simulink model "model_fitting"  (R2019a)
settings: Solver=ode2  StartTime=0.0  StopTime=200  FixedStep=0.1  RelTol=1e-3
settings Model: Creator=HP  LastModifiedBy=swastik
settings DataIOCC: ReturnWorkspaceOutputs=off
settings DebuggingCC: ArithmeticOperatorsInVariantConditions=warning

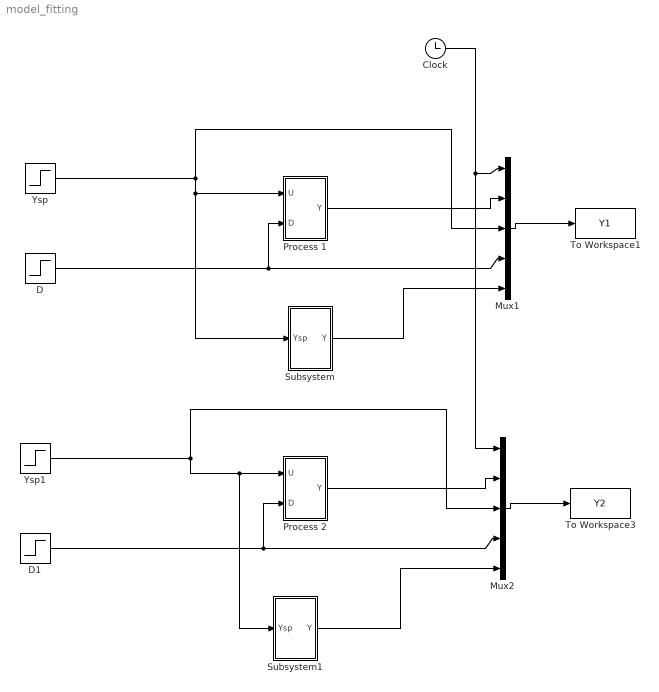
== system model_fitting ==
  Clock : Clock
  D : Step  Time=0  After=0  SampleTime=0
  D1 : Step  Time=0  After=0  SampleTime=0
  Mux1 : Mux  Inputs=5
  Mux2 : Mux  Inputs=5
  Process 1 : Subsystem
  Process 2 : Subsystem
  Subsystem : Subsystem  mask{Km=1.9991, Tm=16.6899, D=23.3484}
      mask prompts: Km "Gain"; Tm "lag"; D "dead time"
  Subsystem1 : Subsystem  mask{K=0.9992, T1=11.25, T2=11.25, T3=15.25, D=16}
      mask prompts: K "Gain1"; T1 "lag1"; T2 "lag2"; T3 "lead"; D "dead time"
  To Workspace1 : ToWorkspace  VariableName=Y1  SampleTime=-1
  To Workspace3 : ToWorkspace  VariableName=Y2  SampleTime=-1
  Ysp : Step  Time=0  SampleTime=0
  Ysp1 : Step  Time=0  SampleTime=0
  wires:
  Mux1/1 -> To Workspace1/1
  Clock/1 -> Mux1/1, Mux2/1
  Ysp/1 -> Subsystem/1(Ysp), Process 1/1(U), Mux1/3
  Process 1/1(Y) -> Mux1/2
  D/1 -> Mux1/4, Process 1/2(D)
  Mux2/1 -> To Workspace3/1
  Ysp1/1 -> Process 2/1(U), Subsystem1/1(Ysp), Mux2/3
  Process 2/1(Y) -> Mux2/2
  D1/1 -> Process 2/2(D), Mux2/4
  Subsystem/1(Y) -> Mux1/5
  Subsystem1/1(Y) -> Mux2/5

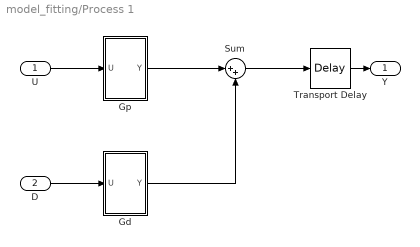
== system model_fitting/Process 1 ==
  U : Inport
  D : Inport  Port=2
  Gd : Subsystem  mask{K1=0.45, K2=0.45, T1=0.3, T2=0.3, K=1/17e-4}
      mask prompts: K1 "Forward Gain"; K2 "Rev Gain"; T1 "Forward Time Constt"; T2 "Rev Time Constt"; K "Scaling Gain"
  Gp : Subsystem  mask{K1=0.45, K2=0.45, T1=0.2, T2=0.2, K=2.01/17e-4}
      mask prompts: K1 "Forward Gain"; K2 "Rev Gain"; T1 "Forward Time Constt"; T2 "Rev Time Constt"; K "Scaling Gain"
  Sum : Sum  Inputs=|++
  Transport Delay : TransportDelay  DelayTime=10
  Y : Outport
  wires:
  Gp/1(Y) -> Sum/1
  Gd/1(Y) -> Sum/2
  D/1 -> Gd/1(U)
  Transport Delay/1 -> Y/1
  Sum/1 -> Transport Delay/1
  U/1 -> Gp/1(U)

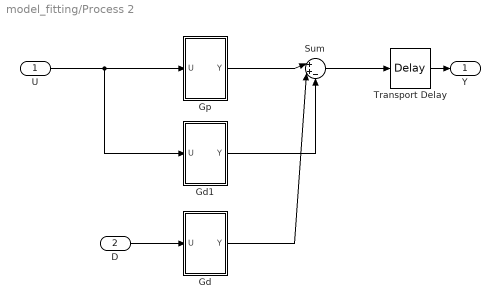
== system model_fitting/Process 2 ==
  U : Inport
  D : Inport  Port=2
  Gd : Subsystem  mask{K1=0.45, K2=0.45, T1=0.3, T2=0.3, K=1/17e-4}
      mask prompts: K1 "Forward Gain"; K2 "Rev Gain"; T1 "Forward Time Constt"; T2 "Rev Time Constt"; K "Scaling Gain"
  Gd1 : Subsystem  mask{K1=0.45, K2=0.45, T1=0.1, T2=0.1, K=1/17e-4}
      mask prompts: K1 "Forward Gain"; K2 "Rev Gain"; T1 "Forward Time Constt"; T2 "Rev Time Constt"; K "Scaling Gain"
  Gp : Subsystem  mask{K1=0.45, K2=0.45, T1=0.2, T2=0.2, K=2.01/17e-4}
      mask prompts: K1 "Forward Gain"; K2 "Rev Gain"; T1 "Forward Time Constt"; T2 "Rev Time Constt"; K "Scaling Gain"
  Sum : Sum  Inputs=|++-
  Transport Delay : TransportDelay  DelayTime=10
  Y : Outport
  wires:
  Gp/1(Y) -> Sum/1
  Gd/1(Y) -> Sum/2
  D/1 -> Gd/1(U)
  Transport Delay/1 -> Y/1
  Sum/1 -> Transport Delay/1
  U/1 -> Gd1/1(U), Gp/1(U)
  Gd1/1(Y) -> Sum/3

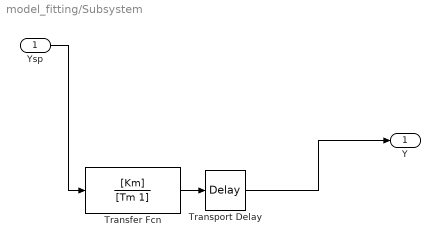
== system model_fitting/Subsystem ==
  Ysp : Inport
  Transfer Fcn : TransferFcn  Numerator=[Km]  Denominator=[Tm 1]
  Transport Delay : TransportDelay  DelayTime=D
  Y : Outport
  wires:
  Transfer Fcn/1 -> Transport Delay/1
  Transport Delay/1 -> Y/1
  Ysp/1 -> Transfer Fcn/1

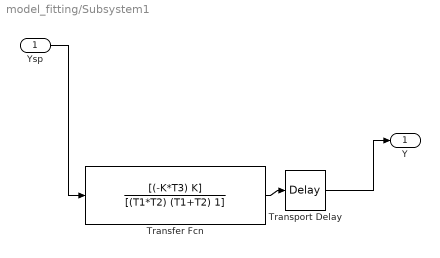
== system model_fitting/Subsystem1 ==
  Ysp : Inport
  Transfer Fcn : TransferFcn  Numerator=[(-K*T3) K]  Denominator=[(T1*T2) (T1+T2) 1]
  Transport Delay : TransportDelay  DelayTime=D
  Y : Outport
  wires:
  Transfer Fcn/1 -> Transport Delay/1
  Ysp/1 -> Transfer Fcn/1
  Transport Delay/1 -> Y/1

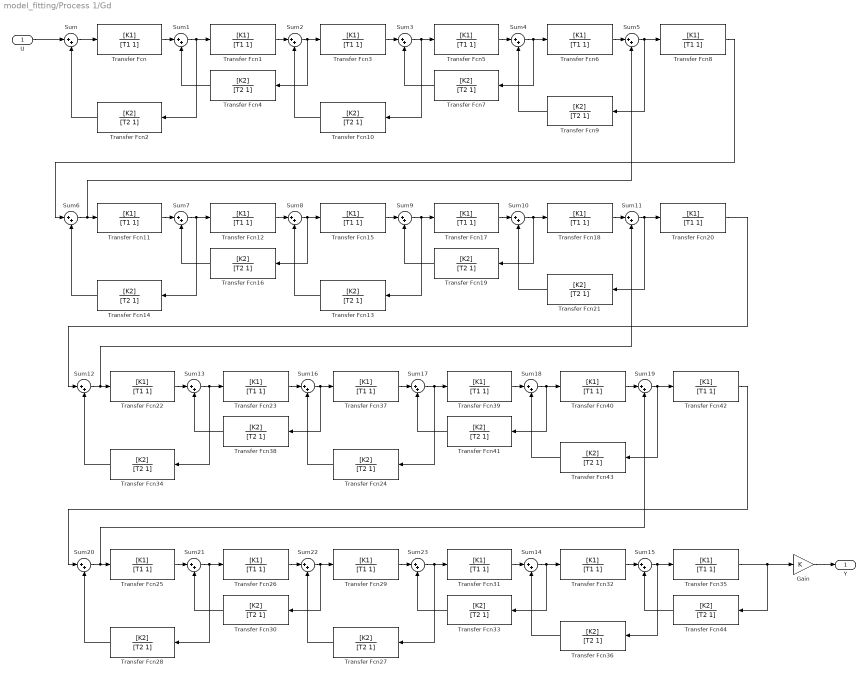
== system model_fitting/Process 1/Gd ==
  U : Inport
  Gain : Gain  Gain=K
  Sum{,1..23} (24 alike) : Sum  Inputs=|++
  Transfer Fcn{,1,3,5..6,8,11..12,15,17..18,20,22..23,25..26,29,31..32,35,37,39..40,42} (24 alike) : TransferFcn  Numerator=[K1]  Denominator=[T1 1]
  Transfer Fcn{2,4,7,9..10,13..14,16,19,21,24,27..28,30,33..34,36,38,41,43..44} (21 alike) : TransferFcn  Numerator=[K2]  Denominator=[T2 1]
  Y : Outport
  wires:
  U/1 -> Sum/1
  Gain/1 -> Y/1
  Sum/1 -> Transfer Fcn/1
  Transfer Fcn19/1 -> Sum9/2
  Transfer Fcn8/1 -> Sum6/1
  Transfer Fcn3/1 -> Sum3/1
  Transfer Fcn10/1 -> Sum2/2
  Transfer Fcn11/1 -> Sum7/1
  Transfer Fcn4/1 -> Sum1/2
  Transfer Fcn7/1 -> Sum3/2
  Sum5/1 -> Transfer Fcn8/1, Transfer Fcn9/1
  Transfer Fcn21/1 -> Sum10/2
  Transfer Fcn/1 -> Sum1/1
  Sum6/1 -> Transfer Fcn11/1, Sum5/2
  Transfer Fcn32/1 -> Sum15/1
  Sum3/1 -> Transfer Fcn5/1, Transfer Fcn10/1
  Sum19/1 -> Transfer Fcn42/1, Transfer Fcn43/1
  Transfer Fcn5/1 -> Sum4/1
  Transfer Fcn43/1 -> Sum18/2
  Transfer Fcn30/1 -> Sum21/2
  Transfer Fcn17/1 -> Sum10/1
  Transfer Fcn28/1 -> Sum20/2
  Transfer Fcn2/1 -> Sum/2
  Transfer Fcn29/1 -> Sum23/1
  Transfer Fcn6/1 -> Sum5/1
  Sum22/1 -> Transfer Fcn29/1, Transfer Fcn30/1
  Sum10/1 -> Transfer Fcn18/1, Transfer Fcn19/1
  Transfer Fcn36/1 -> Sum14/2
  Sum4/1 -> Transfer Fcn6/1, Transfer Fcn7/1
  Transfer Fcn41/1 -> Sum17/2
  Transfer Fcn33/1 -> Sum23/2
  Transfer Fcn37/1 -> Sum17/1
  Transfer Fcn34/1 -> Sum12/2
  Transfer Fcn22/1 -> Sum13/1
  Sum16/1 -> Transfer Fcn37/1, Transfer Fcn38/1
  Transfer Fcn40/1 -> Sum19/1
  Sum23/1 -> Transfer Fcn31/1, Transfer Fcn27/1
  Sum14/1 -> Transfer Fcn32/1, Transfer Fcn33/1
  Transfer Fcn23/1 -> Sum16/1
  Transfer Fcn31/1 -> Sum14/1
  Transfer Fcn24/1 -> Sum16/2
  Transfer Fcn27/1 -> Sum22/2
  Sum15/1 -> Transfer Fcn35/1, Transfer Fcn36/1
  Sum1/1 -> Transfer Fcn1/1, Transfer Fcn2/1
  Transfer Fcn42/1 -> Sum20/1
  Sum11/1 -> Transfer Fcn20/1, Transfer Fcn21/1
  Transfer Fcn35/1 -> Transfer Fcn44/1, Gain/1
  Sum9/1 -> Transfer Fcn17/1, Transfer Fcn13/1
  Sum17/1 -> Transfer Fcn39/1, Transfer Fcn24/1
  Transfer Fcn38/1 -> Sum13/2
  Sum2/1 -> Transfer Fcn3/1, Transfer Fcn4/1
  Transfer Fcn39/1 -> Sum18/1
  Transfer Fcn44/1 -> Sum15/2
  Transfer Fcn16/1 -> Sum7/2
  Transfer Fcn12/1 -> Sum8/1
  Sum12/1 -> Transfer Fcn22/1, Sum11/2
  Transfer Fcn25/1 -> Sum21/1
  Transfer Fcn9/1 -> Sum4/2
  Sum20/1 -> Transfer Fcn25/1, Sum19/2
  Transfer Fcn20/1 -> Sum12/1
  Sum8/1 -> Transfer Fcn15/1, Transfer Fcn16/1
  Sum7/1 -> Transfer Fcn12/1, Transfer Fcn14/1
  Sum13/1 -> Transfer Fcn23/1, Transfer Fcn34/1
  Transfer Fcn15/1 -> Sum9/1
  Transfer Fcn26/1 -> Sum22/1
  Sum21/1 -> Transfer Fcn26/1, Transfer Fcn28/1
  Sum18/1 -> Transfer Fcn40/1, Transfer Fcn41/1
  Transfer Fcn1/1 -> Sum2/1
  Transfer Fcn18/1 -> Sum11/1
  Transfer Fcn13/1 -> Sum8/2
  Transfer Fcn14/1 -> Sum6/2

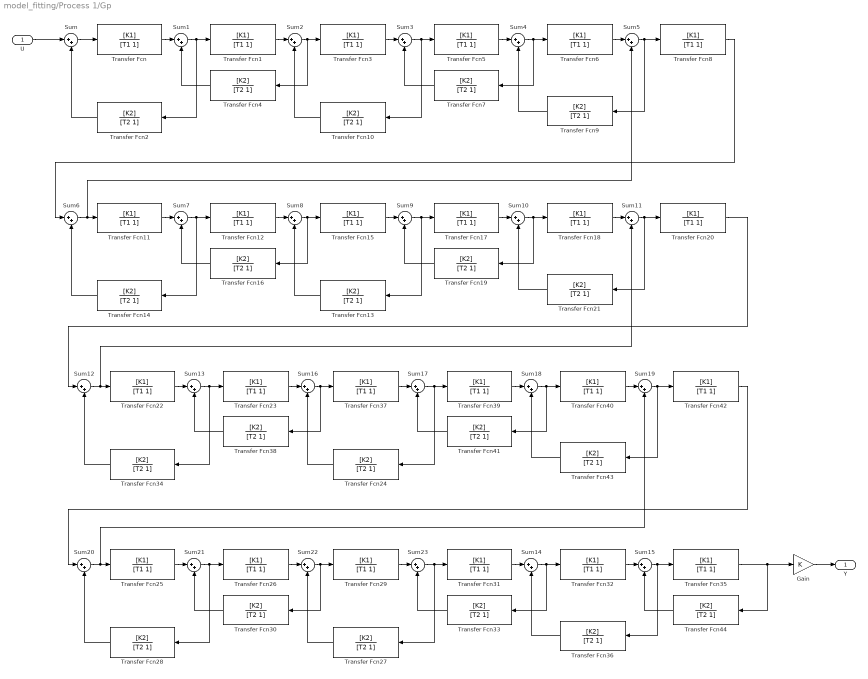
== system model_fitting/Process 1/Gp ==
  U : Inport
  Gain : Gain  Gain=K
  Sum{,1..23} (24 alike) : Sum  Inputs=|++
  Transfer Fcn{,1,3,5..6,8,11..12,15,17..18,20,22..23,25..26,29,31..32,35,37,39..40,42} (24 alike) : TransferFcn  Numerator=[K1]  Denominator=[T1 1]
  Transfer Fcn{2,4,7,9..10,13..14,16,19,21,24,27..28,30,33..34,36,38,41,43..44} (21 alike) : TransferFcn  Numerator=[K2]  Denominator=[T2 1]
  Y : Outport
  wires:
  U/1 -> Sum/1
  Gain/1 -> Y/1
  Sum/1 -> Transfer Fcn/1
  Transfer Fcn19/1 -> Sum9/2
  Transfer Fcn8/1 -> Sum6/1
  Transfer Fcn3/1 -> Sum3/1
  Transfer Fcn10/1 -> Sum2/2
  Transfer Fcn11/1 -> Sum7/1
  Transfer Fcn4/1 -> Sum1/2
  Transfer Fcn7/1 -> Sum3/2
  Sum5/1 -> Transfer Fcn8/1, Transfer Fcn9/1
  Transfer Fcn21/1 -> Sum10/2
  Transfer Fcn/1 -> Sum1/1
  Sum6/1 -> Transfer Fcn11/1, Sum5/2
  Transfer Fcn32/1 -> Sum15/1
  Sum3/1 -> Transfer Fcn5/1, Transfer Fcn10/1
  Sum19/1 -> Transfer Fcn42/1, Transfer Fcn43/1
  Transfer Fcn5/1 -> Sum4/1
  Transfer Fcn43/1 -> Sum18/2
  Transfer Fcn30/1 -> Sum21/2
  Transfer Fcn17/1 -> Sum10/1
  Transfer Fcn28/1 -> Sum20/2
  Transfer Fcn2/1 -> Sum/2
  Transfer Fcn29/1 -> Sum23/1
  Transfer Fcn6/1 -> Sum5/1
  Sum22/1 -> Transfer Fcn29/1, Transfer Fcn30/1
  Sum10/1 -> Transfer Fcn18/1, Transfer Fcn19/1
  Transfer Fcn36/1 -> Sum14/2
  Sum4/1 -> Transfer Fcn6/1, Transfer Fcn7/1
  Transfer Fcn41/1 -> Sum17/2
  Transfer Fcn33/1 -> Sum23/2
  Transfer Fcn37/1 -> Sum17/1
  Transfer Fcn34/1 -> Sum12/2
  Transfer Fcn22/1 -> Sum13/1
  Sum16/1 -> Transfer Fcn37/1, Transfer Fcn38/1
  Transfer Fcn40/1 -> Sum19/1
  Sum23/1 -> Transfer Fcn31/1, Transfer Fcn27/1
  Sum14/1 -> Transfer Fcn32/1, Transfer Fcn33/1
  Transfer Fcn23/1 -> Sum16/1
  Transfer Fcn31/1 -> Sum14/1
  Transfer Fcn24/1 -> Sum16/2
  Transfer Fcn27/1 -> Sum22/2
  Sum15/1 -> Transfer Fcn35/1, Transfer Fcn36/1
  Sum1/1 -> Transfer Fcn1/1, Transfer Fcn2/1
  Transfer Fcn42/1 -> Sum20/1
  Sum11/1 -> Transfer Fcn20/1, Transfer Fcn21/1
  Transfer Fcn35/1 -> Transfer Fcn44/1, Gain/1
  Sum9/1 -> Transfer Fcn17/1, Transfer Fcn13/1
  Sum17/1 -> Transfer Fcn39/1, Transfer Fcn24/1
  Transfer Fcn38/1 -> Sum13/2
  Sum2/1 -> Transfer Fcn3/1, Transfer Fcn4/1
  Transfer Fcn39/1 -> Sum18/1
  Transfer Fcn44/1 -> Sum15/2
  Transfer Fcn16/1 -> Sum7/2
  Transfer Fcn12/1 -> Sum8/1
  Sum12/1 -> Transfer Fcn22/1, Sum11/2
  Transfer Fcn25/1 -> Sum21/1
  Transfer Fcn9/1 -> Sum4/2
  Sum20/1 -> Transfer Fcn25/1, Sum19/2
  Transfer Fcn20/1 -> Sum12/1
  Sum8/1 -> Transfer Fcn15/1, Transfer Fcn16/1
  Sum7/1 -> Transfer Fcn12/1, Transfer Fcn14/1
  Sum13/1 -> Transfer Fcn23/1, Transfer Fcn34/1
  Transfer Fcn15/1 -> Sum9/1
  Transfer Fcn26/1 -> Sum22/1
  Sum21/1 -> Transfer Fcn26/1, Transfer Fcn28/1
  Sum18/1 -> Transfer Fcn40/1, Transfer Fcn41/1
  Transfer Fcn1/1 -> Sum2/1
  Transfer Fcn18/1 -> Sum11/1
  Transfer Fcn13/1 -> Sum8/2
  Transfer Fcn14/1 -> Sum6/2

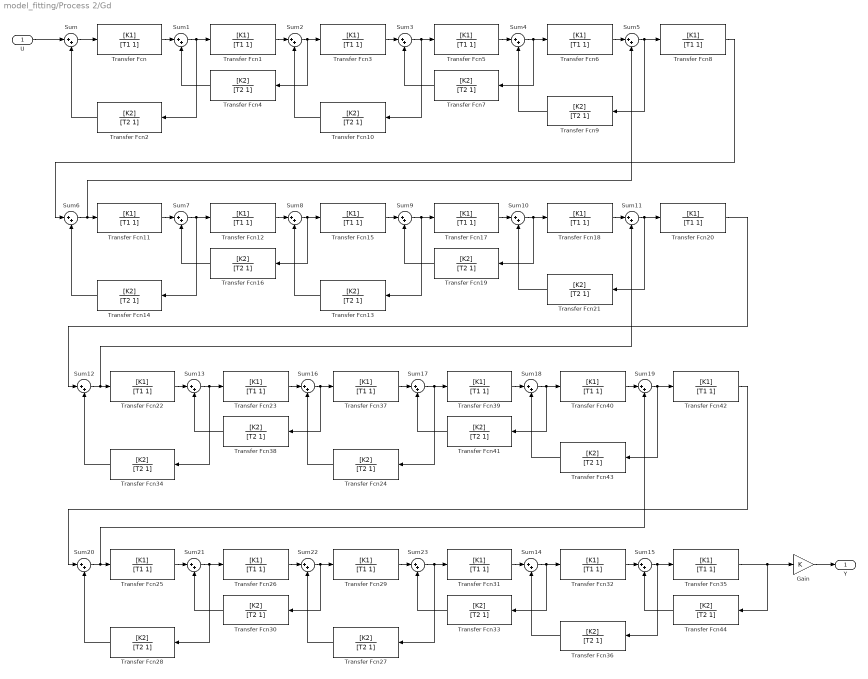
== system model_fitting/Process 2/Gd ==
  U : Inport
  Gain : Gain  Gain=K
  Sum{,1..23} (24 alike) : Sum  Inputs=|++
  Transfer Fcn{,1,3,5..6,8,11..12,15,17..18,20,22..23,25..26,29,31..32,35,37,39..40,42} (24 alike) : TransferFcn  Numerator=[K1]  Denominator=[T1 1]
  Transfer Fcn{2,4,7,9..10,13..14,16,19,21,24,27..28,30,33..34,36,38,41,43..44} (21 alike) : TransferFcn  Numerator=[K2]  Denominator=[T2 1]
  Y : Outport
  wires:
  U/1 -> Sum/1
  Gain/1 -> Y/1
  Sum/1 -> Transfer Fcn/1
  Transfer Fcn19/1 -> Sum9/2
  Transfer Fcn8/1 -> Sum6/1
  Transfer Fcn3/1 -> Sum3/1
  Transfer Fcn10/1 -> Sum2/2
  Transfer Fcn11/1 -> Sum7/1
  Transfer Fcn4/1 -> Sum1/2
  Transfer Fcn7/1 -> Sum3/2
  Sum5/1 -> Transfer Fcn8/1, Transfer Fcn9/1
  Transfer Fcn21/1 -> Sum10/2
  Transfer Fcn/1 -> Sum1/1
  Sum6/1 -> Transfer Fcn11/1, Sum5/2
  Transfer Fcn32/1 -> Sum15/1
  Sum3/1 -> Transfer Fcn5/1, Transfer Fcn10/1
  Sum19/1 -> Transfer Fcn42/1, Transfer Fcn43/1
  Transfer Fcn5/1 -> Sum4/1
  Transfer Fcn43/1 -> Sum18/2
  Transfer Fcn30/1 -> Sum21/2
  Transfer Fcn17/1 -> Sum10/1
  Transfer Fcn28/1 -> Sum20/2
  Transfer Fcn2/1 -> Sum/2
  Transfer Fcn29/1 -> Sum23/1
  Transfer Fcn6/1 -> Sum5/1
  Sum22/1 -> Transfer Fcn29/1, Transfer Fcn30/1
  Sum10/1 -> Transfer Fcn18/1, Transfer Fcn19/1
  Transfer Fcn36/1 -> Sum14/2
  Sum4/1 -> Transfer Fcn6/1, Transfer Fcn7/1
  Transfer Fcn41/1 -> Sum17/2
  Transfer Fcn33/1 -> Sum23/2
  Transfer Fcn37/1 -> Sum17/1
  Transfer Fcn34/1 -> Sum12/2
  Transfer Fcn22/1 -> Sum13/1
  Sum16/1 -> Transfer Fcn37/1, Transfer Fcn38/1
  Transfer Fcn40/1 -> Sum19/1
  Sum23/1 -> Transfer Fcn31/1, Transfer Fcn27/1
  Sum14/1 -> Transfer Fcn32/1, Transfer Fcn33/1
  Transfer Fcn23/1 -> Sum16/1
  Transfer Fcn31/1 -> Sum14/1
  Transfer Fcn24/1 -> Sum16/2
  Transfer Fcn27/1 -> Sum22/2
  Sum15/1 -> Transfer Fcn35/1, Transfer Fcn36/1
  Sum1/1 -> Transfer Fcn1/1, Transfer Fcn2/1
  Transfer Fcn42/1 -> Sum20/1
  Sum11/1 -> Transfer Fcn20/1, Transfer Fcn21/1
  Transfer Fcn35/1 -> Transfer Fcn44/1, Gain/1
  Sum9/1 -> Transfer Fcn17/1, Transfer Fcn13/1
  Sum17/1 -> Transfer Fcn39/1, Transfer Fcn24/1
  Transfer Fcn38/1 -> Sum13/2
  Sum2/1 -> Transfer Fcn3/1, Transfer Fcn4/1
  Transfer Fcn39/1 -> Sum18/1
  Transfer Fcn44/1 -> Sum15/2
  Transfer Fcn16/1 -> Sum7/2
  Transfer Fcn12/1 -> Sum8/1
  Sum12/1 -> Transfer Fcn22/1, Sum11/2
  Transfer Fcn25/1 -> Sum21/1
  Transfer Fcn9/1 -> Sum4/2
  Sum20/1 -> Transfer Fcn25/1, Sum19/2
  Transfer Fcn20/1 -> Sum12/1
  Sum8/1 -> Transfer Fcn15/1, Transfer Fcn16/1
  Sum7/1 -> Transfer Fcn12/1, Transfer Fcn14/1
  Sum13/1 -> Transfer Fcn23/1, Transfer Fcn34/1
  Transfer Fcn15/1 -> Sum9/1
  Transfer Fcn26/1 -> Sum22/1
  Sum21/1 -> Transfer Fcn26/1, Transfer Fcn28/1
  Sum18/1 -> Transfer Fcn40/1, Transfer Fcn41/1
  Transfer Fcn1/1 -> Sum2/1
  Transfer Fcn18/1 -> Sum11/1
  Transfer Fcn13/1 -> Sum8/2
  Transfer Fcn14/1 -> Sum6/2

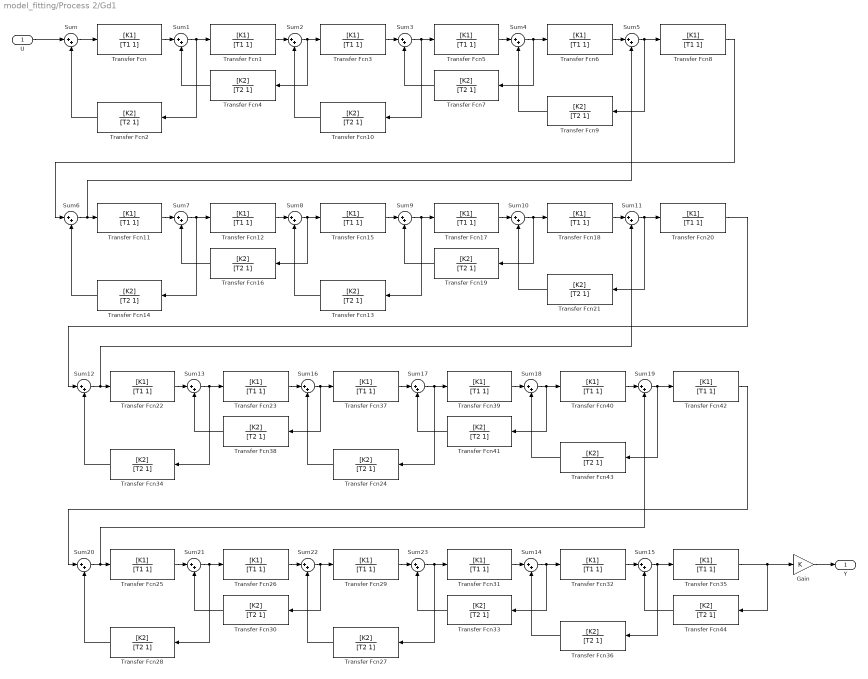
== system model_fitting/Process 2/Gd1 ==
  U : Inport
  Gain : Gain  Gain=K
  Sum{,1..23} (24 alike) : Sum  Inputs=|++
  Transfer Fcn{,1,3,5..6,8,11..12,15,17..18,20,22..23,25..26,29,31..32,35,37,39..40,42} (24 alike) : TransferFcn  Numerator=[K1]  Denominator=[T1 1]
  Transfer Fcn{2,4,7,9..10,13..14,16,19,21,24,27..28,30,33..34,36,38,41,43..44} (21 alike) : TransferFcn  Numerator=[K2]  Denominator=[T2 1]
  Y : Outport
  wires:
  U/1 -> Sum/1
  Gain/1 -> Y/1
  Sum/1 -> Transfer Fcn/1
  Transfer Fcn19/1 -> Sum9/2
  Transfer Fcn8/1 -> Sum6/1
  Transfer Fcn3/1 -> Sum3/1
  Transfer Fcn10/1 -> Sum2/2
  Transfer Fcn11/1 -> Sum7/1
  Transfer Fcn4/1 -> Sum1/2
  Transfer Fcn7/1 -> Sum3/2
  Sum5/1 -> Transfer Fcn8/1, Transfer Fcn9/1
  Transfer Fcn21/1 -> Sum10/2
  Transfer Fcn/1 -> Sum1/1
  Sum6/1 -> Transfer Fcn11/1, Sum5/2
  Transfer Fcn32/1 -> Sum15/1
  Sum3/1 -> Transfer Fcn5/1, Transfer Fcn10/1
  Sum19/1 -> Transfer Fcn42/1, Transfer Fcn43/1
  Transfer Fcn5/1 -> Sum4/1
  Transfer Fcn43/1 -> Sum18/2
  Transfer Fcn30/1 -> Sum21/2
  Transfer Fcn17/1 -> Sum10/1
  Transfer Fcn28/1 -> Sum20/2
  Transfer Fcn2/1 -> Sum/2
  Transfer Fcn29/1 -> Sum23/1
  Transfer Fcn6/1 -> Sum5/1
  Sum22/1 -> Transfer Fcn29/1, Transfer Fcn30/1
  Sum10/1 -> Transfer Fcn18/1, Transfer Fcn19/1
  Transfer Fcn36/1 -> Sum14/2
  Sum4/1 -> Transfer Fcn6/1, Transfer Fcn7/1
  Transfer Fcn41/1 -> Sum17/2
  Transfer Fcn33/1 -> Sum23/2
  Transfer Fcn37/1 -> Sum17/1
  Transfer Fcn34/1 -> Sum12/2
  Transfer Fcn22/1 -> Sum13/1
  Sum16/1 -> Transfer Fcn37/1, Transfer Fcn38/1
  Transfer Fcn40/1 -> Sum19/1
  Sum23/1 -> Transfer Fcn31/1, Transfer Fcn27/1
  Sum14/1 -> Transfer Fcn32/1, Transfer Fcn33/1
  Transfer Fcn23/1 -> Sum16/1
  Transfer Fcn31/1 -> Sum14/1
  Transfer Fcn24/1 -> Sum16/2
  Transfer Fcn27/1 -> Sum22/2
  Sum15/1 -> Transfer Fcn35/1, Transfer Fcn36/1
  Sum1/1 -> Transfer Fcn1/1, Transfer Fcn2/1
  Transfer Fcn42/1 -> Sum20/1
  Sum11/1 -> Transfer Fcn20/1, Transfer Fcn21/1
  Transfer Fcn35/1 -> Transfer Fcn44/1, Gain/1
  Sum9/1 -> Transfer Fcn17/1, Transfer Fcn13/1
  Sum17/1 -> Transfer Fcn39/1, Transfer Fcn24/1
  Transfer Fcn38/1 -> Sum13/2
  Sum2/1 -> Transfer Fcn3/1, Transfer Fcn4/1
  Transfer Fcn39/1 -> Sum18/1
  Transfer Fcn44/1 -> Sum15/2
  Transfer Fcn16/1 -> Sum7/2
  Transfer Fcn12/1 -> Sum8/1
  Sum12/1 -> Transfer Fcn22/1, Sum11/2
  Transfer Fcn25/1 -> Sum21/1
  Transfer Fcn9/1 -> Sum4/2
  Sum20/1 -> Transfer Fcn25/1, Sum19/2
  Transfer Fcn20/1 -> Sum12/1
  Sum8/1 -> Transfer Fcn15/1, Transfer Fcn16/1
  Sum7/1 -> Transfer Fcn12/1, Transfer Fcn14/1
  Sum13/1 -> Transfer Fcn23/1, Transfer Fcn34/1
  Transfer Fcn15/1 -> Sum9/1
  Transfer Fcn26/1 -> Sum22/1
  Sum21/1 -> Transfer Fcn26/1, Transfer Fcn28/1
  Sum18/1 -> Transfer Fcn40/1, Transfer Fcn41/1
  Transfer Fcn1/1 -> Sum2/1
  Transfer Fcn18/1 -> Sum11/1
  Transfer Fcn13/1 -> Sum8/2
  Transfer Fcn14/1 -> Sum6/2

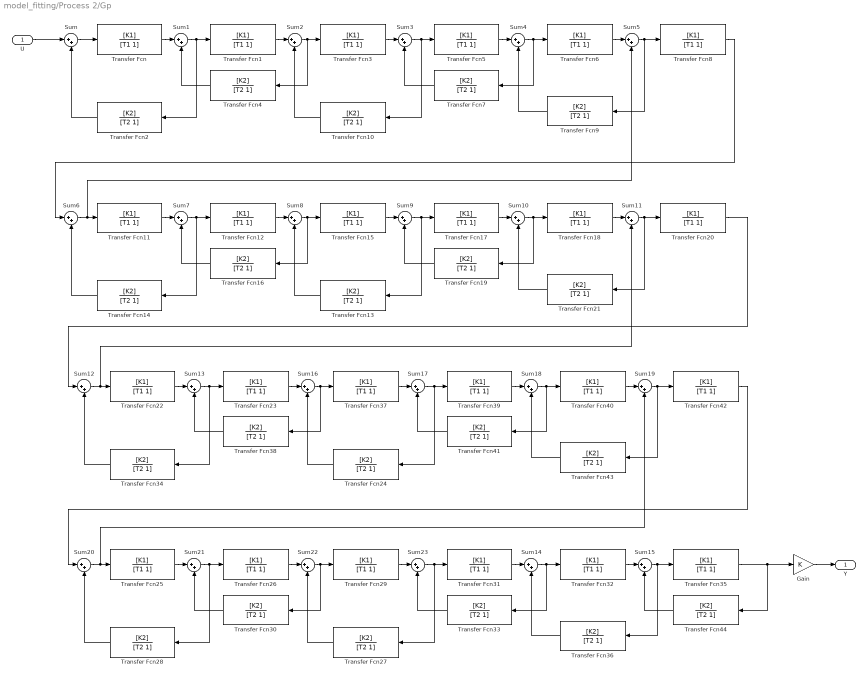
== system model_fitting/Process 2/Gp ==
  U : Inport
  Gain : Gain  Gain=K
  Sum{,1..23} (24 alike) : Sum  Inputs=|++
  Transfer Fcn{,1,3,5..6,8,11..12,15,17..18,20,22..23,25..26,29,31..32,35,37,39..40,42} (24 alike) : TransferFcn  Numerator=[K1]  Denominator=[T1 1]
  Transfer Fcn{2,4,7,9..10,13..14,16,19,21,24,27..28,30,33..34,36,38,41,43..44} (21 alike) : TransferFcn  Numerator=[K2]  Denominator=[T2 1]
  Y : Outport
  wires:
  U/1 -> Sum/1
  Gain/1 -> Y/1
  Sum/1 -> Transfer Fcn/1
  Transfer Fcn19/1 -> Sum9/2
  Transfer Fcn8/1 -> Sum6/1
  Transfer Fcn3/1 -> Sum3/1
  Transfer Fcn10/1 -> Sum2/2
  Transfer Fcn11/1 -> Sum7/1
  Transfer Fcn4/1 -> Sum1/2
  Transfer Fcn7/1 -> Sum3/2
  Sum5/1 -> Transfer Fcn8/1, Transfer Fcn9/1
  Transfer Fcn21/1 -> Sum10/2
  Transfer Fcn/1 -> Sum1/1
  Sum6/1 -> Transfer Fcn11/1, Sum5/2
  Transfer Fcn32/1 -> Sum15/1
  Sum3/1 -> Transfer Fcn5/1, Transfer Fcn10/1
  Sum19/1 -> Transfer Fcn42/1, Transfer Fcn43/1
  Transfer Fcn5/1 -> Sum4/1
  Transfer Fcn43/1 -> Sum18/2
  Transfer Fcn30/1 -> Sum21/2
  Transfer Fcn17/1 -> Sum10/1
  Transfer Fcn28/1 -> Sum20/2
  Transfer Fcn2/1 -> Sum/2
  Transfer Fcn29/1 -> Sum23/1
  Transfer Fcn6/1 -> Sum5/1
  Sum22/1 -> Transfer Fcn29/1, Transfer Fcn30/1
  Sum10/1 -> Transfer Fcn18/1, Transfer Fcn19/1
  Transfer Fcn36/1 -> Sum14/2
  Sum4/1 -> Transfer Fcn6/1, Transfer Fcn7/1
  Transfer Fcn41/1 -> Sum17/2
  Transfer Fcn33/1 -> Sum23/2
  Transfer Fcn37/1 -> Sum17/1
  Transfer Fcn34/1 -> Sum12/2
  Transfer Fcn22/1 -> Sum13/1
  Sum16/1 -> Transfer Fcn37/1, Transfer Fcn38/1
  Transfer Fcn40/1 -> Sum19/1
  Sum23/1 -> Transfer Fcn31/1, Transfer Fcn27/1
  Sum14/1 -> Transfer Fcn32/1, Transfer Fcn33/1
  Transfer Fcn23/1 -> Sum16/1
  Transfer Fcn31/1 -> Sum14/1
  Transfer Fcn24/1 -> Sum16/2
  Transfer Fcn27/1 -> Sum22/2
  Sum15/1 -> Transfer Fcn35/1, Transfer Fcn36/1
  Sum1/1 -> Transfer Fcn1/1, Transfer Fcn2/1
  Transfer Fcn42/1 -> Sum20/1
  Sum11/1 -> Transfer Fcn20/1, Transfer Fcn21/1
  Transfer Fcn35/1 -> Transfer Fcn44/1, Gain/1
  Sum9/1 -> Transfer Fcn17/1, Transfer Fcn13/1
  Sum17/1 -> Transfer Fcn39/1, Transfer Fcn24/1
  Transfer Fcn38/1 -> Sum13/2
  Sum2/1 -> Transfer Fcn3/1, Transfer Fcn4/1
  Transfer Fcn39/1 -> Sum18/1
  Transfer Fcn44/1 -> Sum15/2
  Transfer Fcn16/1 -> Sum7/2
  Transfer Fcn12/1 -> Sum8/1
  Sum12/1 -> Transfer Fcn22/1, Sum11/2
  Transfer Fcn25/1 -> Sum21/1
  Transfer Fcn9/1 -> Sum4/2
  Sum20/1 -> Transfer Fcn25/1, Sum19/2
  Transfer Fcn20/1 -> Sum12/1
  Sum8/1 -> Transfer Fcn15/1, Transfer Fcn16/1
  Sum7/1 -> Transfer Fcn12/1, Transfer Fcn14/1
  Sum13/1 -> Transfer Fcn23/1, Transfer Fcn34/1
  Transfer Fcn15/1 -> Sum9/1
  Transfer Fcn26/1 -> Sum22/1
  Sum21/1 -> Transfer Fcn26/1, Transfer Fcn28/1
  Sum18/1 -> Transfer Fcn40/1, Transfer Fcn41/1
  Transfer Fcn1/1 -> Sum2/1
  Transfer Fcn18/1 -> Sum11/1
  Transfer Fcn13/1 -> Sum8/2
  Transfer Fcn14/1 -> Sum6/2
